simulink model "Buck_Converter_Simulation"  (R2017a)
settings: Solver=FixedStepAuto  StartTime=0.0  StopTime=0.01  FixedStep=1e-8  MaxStep=1e-4  RelTol=1e-3
libraries: powerlib x16, powerlib_meascontrol x1
settings Model: Creator=tunay  LastModifiedBy=user
settings OptimizationCC: LifeSpan=inf
settings DebuggingCC: SFExecutionAtInitializationDiag=none

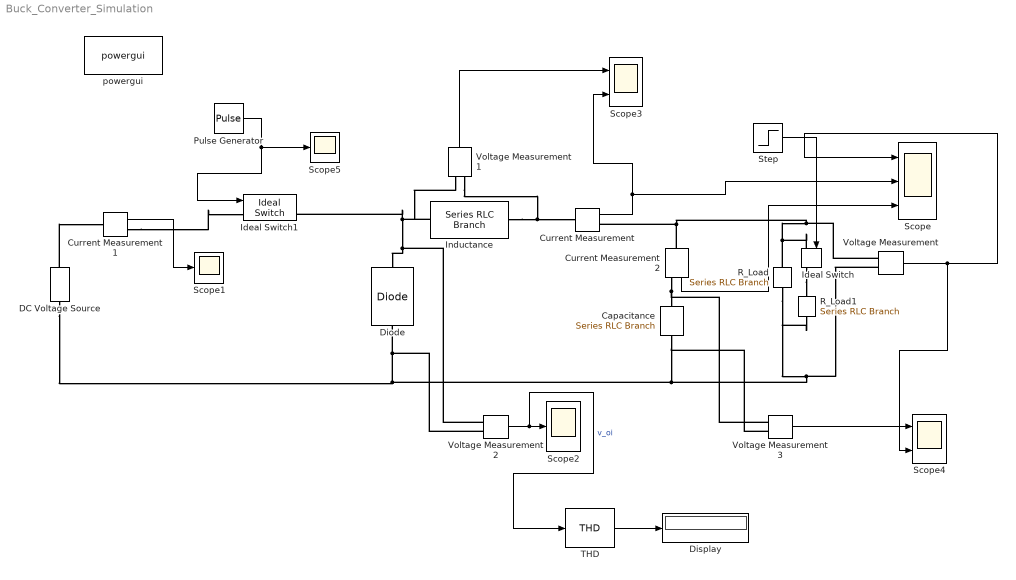
== system Buck_Converter_Simulation ==
  Capacitance : powerlib/Elements/Series RLC Branch  LConnTagsString=__new0  RConnTagsString=__new0  BranchType=RC  Resistance=0.1  Inductance=1e-3  SetiL0=off  InitialCurrent=0  Capacitance=100e-6  Setx0=off  InitialVoltage=0  Measurements=None
  Current Measurement : powerlib/Measurements/Current Measurement  PhasorSimulation=off  OutputType=Complex  PSBequivalent=0
  Current Measurement1 : powerlib/Measurements/Current Measurement  PhasorSimulation=off  OutputType=Complex  PSBequivalent=0
  Current Measurement2 : powerlib/Measurements/Current Measurement  PhasorSimulation=off  OutputType=Complex  PSBequivalent=0
  DC Voltage Source : powerlib/Electrical Sources/DC Voltage Source  Amplitude=8  Measurements=None
  Diode : powerlib/Power Electronics/Diode  Ron=0.001  Lon=0  Vf=0.8  IC=0  UseSnubber=0  Rs=500  Cs=1e-12  Measurements=off
  Display : Display
  Ideal Switch : powerlib/Power Electronics/Ideal Switch  Ron=1e-10  Lon=0  IC=1  Rs=inf  Cs=0  Measurements=on
  Ideal Switch1 : powerlib/Power Electronics/Ideal Switch  Ron=1e-10  Lon=0  IC=1  Rs=inf  Cs=0  Measurements=on
  Inductance : powerlib/Elements/Series RLC Branch  LConnTagsString=__new0  RConnTagsString=__new0  BranchType=L  Resistance=10e-3  Inductance=10e-6  SetiL0=off  InitialCurrent=0  Capacitance=1e-6  Setx0=off  InitialVoltage=0  Measurements=None
  Pulse Generator : DiscretePulseGenerator  PulseType=Time based  Period=1/50000  PulseWidth=75
  R_Load : powerlib/Elements/Series RLC Branch  LConnTagsString=__new0  RConnTagsString=__new0  BranchType=R  Resistance=10  Inductance=200e-6  SetiL0=off  InitialCurrent=0  Capacitance=1e-6  Setx0=off  InitialVoltage=0  Measurements=None
  R_Load1 : powerlib/Elements/Series RLC Branch  LConnTagsString=__new0  RConnTagsString=__new0  BranchType=R  Resistance=10/19  Inductance=200e-6  SetiL0=off  InitialCurrent=0  Capacitance=1e-6  Setx0=off  InitialVoltage=0  Measurements=None
  Scope : Scope  NumInputPorts=3
  Scope1 : Scope
  Scope2 : Scope
  Scope3 : Scope  NumInputPorts=2
  Scope4 : Scope  NumInputPorts=2
  Scope5 : Scope
  Step : Step  Time=0.005  Before=1  SampleTime=0
  THD : powerlib_meascontrol/Measurements/THD  Freq=50000  Ts=1e-8
  Voltage Measurement{,1..3} (4 alike) : powerlib/Measurements/Voltage Measurement  PhasorSimulation=off  OutputType=Complex  PSBequivalent=0
  powergui : powerlib/powergui  Priority=1  SimulationMode=Discrete  SampleTime=1e-8  frequency=60  Iterations=50  frequencyindice=0  Pbase=100e6  ErrMax=1e-4  UnitsV=kV  UnitsW=MW  buscounter=0  FunctionMessages=off  echomessages=off  EnableUseOfTLC=off  CurrentSourceSwitches=off  DisableSnubberDevices=off  DisableRonSwitches=off  DisableVfSwitches=off  DisplayEquations=off  SolverType=Tustin/Backward Euler (TBE)  Interpol=off  ExternalGateDelay=off  methode=off  Ts=100  x0status=blocks  SPID=off  SwTol=0  HookPort=off  RestoreLinks=warning  ResistiveCurrentMeasurement=off  Frange=[0:2:500]  Ylog=off  Xlog=on  ShowGrid=off  save=off  variable=ZData  structure=logsout  ZoomFFT=off  StartTime=0.0002  cycles=20  DisplayStyle=1  fundamental=50000  FreqAxis=on  MaxFrequency=1200000  frequencyindicesteady=1  RmsSteady=1  display=off
  wires:
  Pulse Generator/1 -> Ideal Switch1/1, Scope5/1
  Current Measurement1/1 -> Scope1/1
  Voltage Measurement/1 -> Scope4/2, Scope/1
  Current Measurement/1 -> Scope/2, Scope3/2
  Voltage Measurement1/1 -> Scope3/1
  Voltage Measurement2/1 -> THD/1, Scope2/1  "v_oi"
  Current Measurement2/1 -> Scope/3
  Voltage Measurement3/1 -> Scope4/1
  THD/1 -> Display/1
  Step/1 -> Ideal Switch/1
  connections:
  DC Voltage Source/LConn1 -- Voltage Measurement3/LConn2 -- Capacitance/RConn1 -- R_Load1/RConn1 -- R_Load/RConn1 -- Voltage Measurement/LConn2 -- Voltage Measurement2/LConn2 -- Diode/LConn1
  R_Load/LConn1 -- Ideal Switch/LConn1 -- Voltage Measurement/LConn1 -- Current Measurement2/LConn1 -- Current Measurement/RConn1
  Inductance/RConn1 -- Voltage Measurement1/LConn2 -- Current Measurement/LConn1
  Current Measurement1/RConn1 -- Ideal Switch1/LConn1
  DC Voltage Source/RConn1 -- Current Measurement1/LConn1
  Current Measurement2/RConn1 -- Voltage Measurement3/LConn1 -- Capacitance/LConn1
  Ideal Switch/RConn1 -- R_Load1/LConn1
  Voltage Measurement1/LConn1 -- Inductance/LConn1 -- Ideal Switch1/RConn1 -- Voltage Measurement2/LConn1 -- Diode/RConn1
